simulink model "EXERCICE_2"  (R2020a)
settings: Solver=VariableStepAuto  StartTime=0.0  StopTime=20  RelTol=1e-3
libraries: cstblocks x13
settings Model: Creator=mehdi  LastModifiedBy=mehdi

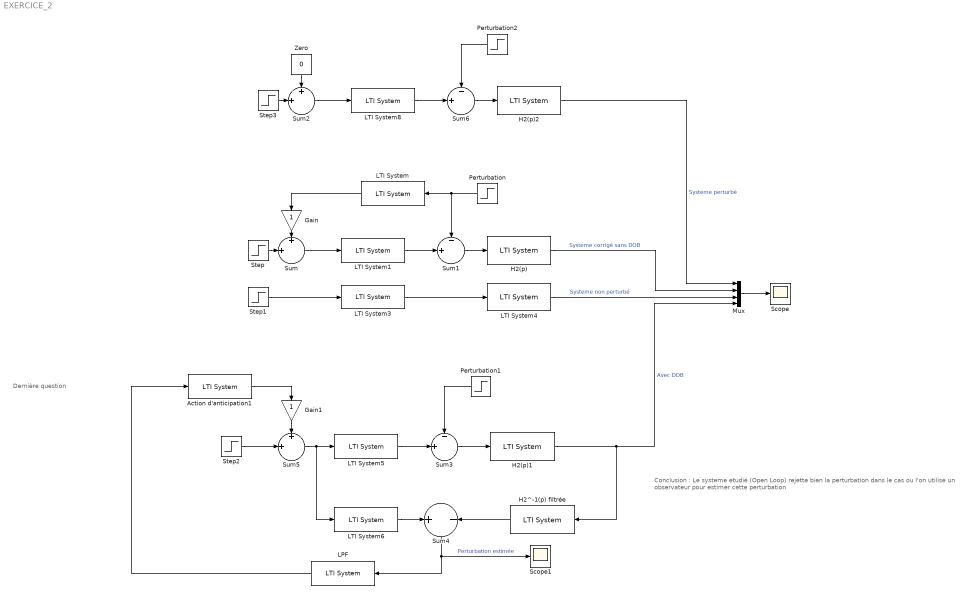
== system EXERCICE_2 ==
  note: Conclusion : Le systeme etudié (Open Loop) rejette bien la perturbation
      | dans le cas ou l'on utilise un observateur pour estimer cette perturbation
  note: Dernière question
  Action d'anticipation1 : cstblocks/LTI System  sys=G  IC=[]
  Gain : Gain
  Gain1 : Gain
  H2(p) : cstblocks/LTI System  sys=H2  IC=[]
  H2(p)1 : cstblocks/LTI System  sys=H2  IC=[]
  H2(p)2 : cstblocks/LTI System  sys=H2  IC=[]
  H2^-1(p) filtrée : cstblocks/LTI System  sys=H2_inv  IC=[]
  LPF : cstblocks/LTI System  sys=Q  IC=[]
  LTI System : cstblocks/LTI System  sys=G  IC=[]
  LTI System{1,3,5..6,8} (5 alike) : cstblocks/LTI System  sys=H1  IC=[]
  LTI System4 : cstblocks/LTI System  sys=H2  IC=[]
  Mux : Mux
  Perturbation : Step  Time=3.5  After=2.45  SampleTime=0
  Perturbation1 : Step  Time=3.5  After=2.45  SampleTime=0
  Perturbation2 : Step  Time=3.5  After=2.45  SampleTime=0
  Scope : Scope
  Scope1 : Scope
  Step{,1..3} (4 alike) : Step  Time=0  SampleTime=0
  Sum : Sum  Inputs=+||+|||
  Sum1 : Sum  Inputs=-||+|||
  Sum2 : Sum  Inputs=+||+|||
  Sum3 : Sum  Inputs=-||+|||
  Sum4 : Sum  Inputs=+||||-
  Sum5 : Sum  Inputs=+||+|||
  Sum6 : Sum  Inputs=-||+|||
  Zero : Constant  Value=0  OutDataTypeStr=Inherit: Inherit via back propagation
  wires:
  Step/1 -> Sum/2
  Perturbation/1 -> LTI System/1, Sum1/1
  Gain/1 -> Sum/1
  LTI System/1 -> Gain/1
  Sum/1 -> LTI System1/1
  LTI System1/1 -> Sum1/2
  H2(p)/1 -> Mux/2  "Systeme corrigé sans DOB"
  Sum1/1 -> H2(p)/1
  Step1/1 -> LTI System3/1
  LTI System3/1 -> LTI System4/1
  LTI System4/1 -> Mux/3  "Systeme non perturbé"
  Gain1/1 -> Sum5/1
  Step2/1 -> Sum5/2
  Perturbation1/1 -> Sum3/1
  LTI System5/1 -> Sum3/2
  Sum5/1 -> LTI System5/1, LTI System6/1
  LPF/1 -> Action d'anticipation1/1
  H2(p)1/1 -> Mux/4, H2^-1(p) filtrée/1  "Avec DOB"
  Sum3/1 -> H2(p)1/1
  LTI System6/1 -> Sum4/1
  H2^-1(p) filtrée/1 -> Sum4/2
  Mux/1 -> Scope/1
  Sum4/1 -> LPF/1, Scope1/1  "Perturbation estimée"
  H2(p)2/1 -> Mux/1  "Systeme perturbé"
  Step3/1 -> Sum2/2
  Perturbation2/1 -> Sum6/1
  LTI System8/1 -> Sum6/2
  Sum2/1 -> LTI System8/1
  Sum6/1 -> H2(p)2/1
  Zero/1 -> Sum2/1
  Action d'anticipation1/1 -> Gain1/1
